simulink model "punkt4"  (R2015b)
settings: Solver=VariableStepAuto  StartTime=0.0  StopTime=10  RelTol=1e-3
settings Model: Creator=hohotulca  LastModifiedBy=hohotulca

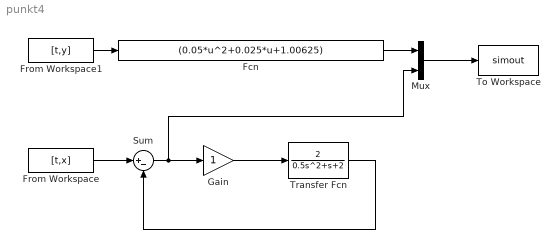
== system punkt4 ==
  Fcn : Fcn  Expr=(0.05*u^2+0.025*u+1.00625)
  From Workspace : FromWorkspace  VariableName=[t,x]  SampleTime=0
  From Workspace1 : FromWorkspace  VariableName=[t,y]  SampleTime=0
  Gain : Gain
  Mux : Mux  Inputs=2
  Sum : Sum  Inputs=|+-
  To Workspace : ToWorkspace  VariableName=simout  SaveFormat=Timeseries  SampleTime=-1
  Transfer Fcn : TransferFcn  Numerator=[ 2]  Denominator=[0.5 1 2]
  wires:
  Transfer Fcn/1 -> Sum/2
  From Workspace/1 -> Sum/1
  Sum/1 -> Mux/2, Gain/1
  Gain/1 -> Transfer Fcn/1
  From Workspace1/1 -> Fcn/1
  Mux/1 -> To Workspace/1
  Fcn/1 -> Mux/1
